simulink model "Sim_Part10_and_11"  (R2017b)
settings: Solver=VariableStepAuto  StartTime=0.0  StopTime=100  RelTol=1e-3
settings Model: Creator=Mohammadreza  LastModifiedBy=Mohammadreza

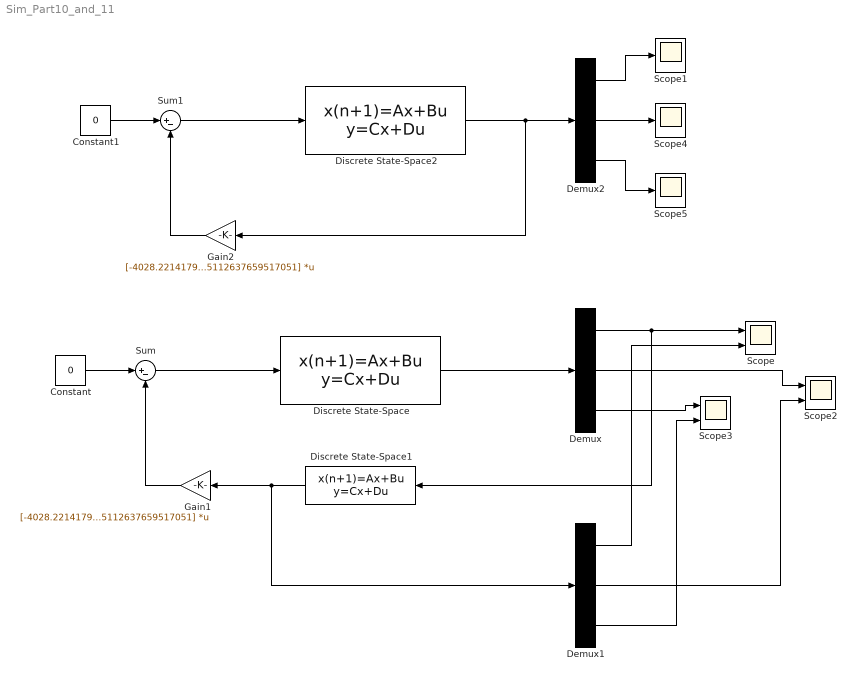
== system Sim_Part10_and_11 ==
  Constant : Constant  Value=0
  Constant1 : Constant  Value=0
  Demux : Demux  Outputs=3
  Demux1 : Demux  Outputs=3
  Demux2 : Demux  Outputs=3
  Discrete State-Space : DiscreteStateSpace  A="[1, -17.129264753527277065, -0.00040142976010392264225; 0, 0.90483741803595951758, 0.000041247798654724229708; 0, 0,  0.69119497372174687477]"  B=|  C=[1 0 0; 0 1 0; 0 0 1]  D=[0; 0; 0]  InitialCondition=[1, 1, 1]  SampleTime=4
      | [-0.000046347083088351534216;
      | 0.0000074338844463689355629; 0.27870489736304436955]
  Discrete State-Space1 : DiscreteStateSpace  A="[-1.7827287045119768348,   -11.099346634521331398,  -0.00016160625662055117703; 0.12967896576651363365, -0.062337030295668631434, 0.0000027810798534536567168; 1654.6249503650512645,   -36260.484985893161207,     -0.75096665695005970679]"  B=[2.5960323917577055042; -0.099733633221363124366; -531.9399135301100614]  C=[1 0 0; 0 1 0; 0 0 1]  D=[0; 0; 0]  SampleTime=-1
  Discrete State-Space2 : DiscreteStateSpace  A="[1, -17.129264753527277065, -0.00040142976010392264225; 0, 0.90483741803595951758, 0.000041247798654724229708; 0, 0,  0.69119497372174687477]"  B=|  C=[1 0 0; 0 1 0; 0 0 1]  D=[0; 0; 0]  InitialCondition=[1, 1, 1]  SampleTime=4
      | [-0.000046347083088351534216;
      | 0.0000074338844463689355629; 0.27870489736304436955]
  Gain1 : Gain  Gain=[-4028.2214179125747402, 130103.50851014941077, 5.1745112637659517051]  Multiplication=Matrix(K*u)
  Gain2 : Gain  Gain=[-4028.2214179125747402, 130103.50851014941077, 5.1745112637659517051]  Multiplication=Matrix(K*u)
  Scope : Scope  NumInputPorts=2
  Scope1 : Scope
  Scope2 : Scope  NumInputPorts=2
  Scope3 : Scope  NumInputPorts=2
  Scope4 : Scope
  Scope5 : Scope
  Sum : Sum  Inputs=|+-
  Sum1 : Sum  Inputs=|+-
  wires:
  Constant/1 -> Sum/1
  Sum/1 -> Discrete State-Space/1
  Discrete State-Space/1 -> Demux/1
  Demux/1 -> Discrete State-Space1/1, Scope/1
  Gain1/1 -> Sum/2
  Demux/2 -> Scope2/1
  Demux/3 -> Scope3/1
  Discrete State-Space1/1 -> Demux1/1, Gain1/1
  Demux1/1 -> Scope/2
  Demux1/2 -> Scope2/2
  Demux1/3 -> Scope3/2
  Demux2/3 -> Scope5/1
  Demux2/1 -> Scope1/1
  Constant1/1 -> Sum1/1
  Gain2/1 -> Sum1/2
  Sum1/1 -> Discrete State-Space2/1
  Discrete State-Space2/1 -> Gain2/1, Demux2/1
  Demux2/2 -> Scope4/1
